simulink model "satellite_ADCS_pointing_simulation"  (R2022b)
settings: Solver=FixedStepAuto  StartTime=t0  StopTime=T_o  FixedStep=0.1  RelTol=1e-9  AbsTol=1e-9
values from neighbouring files (symbols this model uses):
  A0 = Af    [satellite_ADCS_LEOP_simulation.m]
  a0 = [adx0 ady0 adz0 ax0 ay0 az0]    [satellite_ADCS_LEOP_simulation.m]
  A_sb_1 = [999.999999992226e-003    3.46376307675883e-006   -1.88420189887425e-006 ... (first row only)    [satellite_ADCS_LEOP_simulation.m]
  A_sb_2 = [999.999999948501e-003   -10.1488410044293e-006   -22.0178875132149e-012 ... (first row only)    [satellite_ADCS_LEOP_simulation.m]
  A_sb_3 = [999.999999975613e-003   -46.6812699606578e-012    6.98384920637069e-006 ... (first row only)    [satellite_ADCS_LEOP_simulation.m]
  Ac = [0 (1-Ky)*n 0 -Ky*n^2 0 0 ... (first row only)    [satellite_ADCS_LEOP_simulation.m]
  alphaG_0 = pi/1.5    (= 2.09439510239)    [satellite_ADCS_LEOP_simulation.m]
  Bc = [J^-1; zeros(3,3)]    [satellite_ADCS_LEOP_simulation.m]
  Cc = [0 0 0 1 0 0 ... (first row only)    [satellite_ADCS_LEOP_simulation.m]
  Dc = zeros(3,3)    [satellite_ADCS_LEOP_simulation.m]
  E = 1    [satellite_ADCS_LEOP_simulation.m]
  F = 1e-3    (= 0.001)    [satellite_ADCS_LEOP_simulation.m]
  FOV = deg2rad(21.7)    [satellite_ADCS_LEOP_simulation.m]
  g_nm = S_matrix.*g_coefficients    [satellite_ADCS_LEOP_simulation.m]
  h_nm = S_matrix.*h_coefficients    [satellite_ADCS_LEOP_simulation.m]
  J = diag([Ix,Iy,Iz])    [satellite_ADCS_LEOP_simulation.m]
  J2 = 1.082e-3    (= 0.001082)    [satellite_ADCS_LEOP_simulation.m]
  K = lqry(SC,Qc,Rc)    [satellite_ADCS_LEOP_simulation.m]
  K_matrix = zeros(5,6)    [satellite_ADCS_LEOP_simulation.m]
  kep = [a e i OM om thf]    [satellite_ADCS_LEOP_simulation.m]
  L = Lt'    [satellite_ADCS_LEOP_simulation.m]
  LL = 1e-5    (= 1e-05)    [satellite_ADCS_LEOP_simulation.m]
  m = [0.37 0.32 0.28]    [satellite_ADCS_LEOP_simulation.m]
  mu = astroConstants(13)    [satellite_ADCS_LEOP_simulation.m]
  n_sun = 2*pi/T_y    (= 1.99238499086e-07)    [satellite_ADCS_LEOP_simulation.m]
  omega_e = 2*pi/T_e    (= 7.27220521664e-05)    [satellite_ADCS_LEOP_simulation.m]
  P00 = 1    [satellite_ADCS_LEOP_simulation.m]
  pR = pinv(R)    [satellite_ADCS_LEOP_simulation.m]
  R = [0 0 dz/2 0 0 -dz/2 ... (first row only)    [satellite_ADCS_LEOP_simulation.m]
  rt = astroConstants(23)    [satellite_ADCS_LEOP_simulation.m]
  S = S'    [satellite_ADCS_LEOP_simulation.m]
  sensor_noise = deg2rad(50/3600)    [satellite_ADCS_LEOP_simulation.m]
  sensor_sample_time = 1    [satellite_ADCS_LEOP_simulation.m]
  t0 = tf    (= 3200)    [satellite_ADCS_LEOP_simulation.m]
  T_o = 2*pi/n    [satellite_ADCS_LEOP_simulation.m]
  Te = 0.03    [satellite_ADCS_LEOP_simulation.m]
  Tp = [999.999926226686e-003    355.891478141766e-006   -144.526391847740e-006 ... (first row only)    [satellite_ADCS_LEOP_simulation.m]
  UL = 1e-4    (= 0.0001)    [satellite_ADCS_LEOP_simulation.m]
  w0 = wf    [satellite_ADCS_LEOP_simulation.m]
libraries: matrix_library x7, vrlib x3, sharedutil x2, aerolibutil x2
(part 2 of 3)

== system satellite_ADCS_pointing_simulation/SAD/Attitude Determination ==
  note: matrix of star catalogue in inertial frame
  note: Star Sampling & Attitude Determination
  note: s/c attitude
  S_n : Inport
  w : Inport  Port=2
  A_b/n : Inport  Port=3
  Algebraic Attitude Determination : Subsystem  Commented=on
      settings: PortSchema="{\"entries\":[{\"content\":{\"sides\":[{\"content\":{\"connectorIds\":[\"In1\",\"In2\"]},\"type\":\"ConnectorPlacement.EquallySpacedRectSide\",\"uuid\":\"6504138f-2a85-4d38-9815-f5cddec5de59\"},{\"content\":{\"connectorIds\":[\"Out1\"],\"side\":\"RIGHT\"},\"type\":\"ConnectorPlacement.EquallySpacedRectSide\",\"uuid\":\"322c0af4-c8eb-4770-b746-148ad674ab50\"},{\"content\":{\"connectorIds\":[\"In3\"],\"side\":\"TOP\"},\"type\":\"ConnectorPlacement.EquallySpacedRectSide\",\"uuid\":\"b986788c-e235-4c96-906b-8e6936550346\"}]},\"type\":\"ConnectorPlacement.EquallySpacedConnector\",\"uuid\":\"9dab80e4-0566-4f6e-b7d4-73f1fb3580cf\"}],\"packageUris\":[\"http://schema.mathworks.com/mf0/Connector/R2020b\"],\"version\":\"1.0\"}"
  Constant3 : Constant  Value=S
  Demux : Demux  Outputs=3
  Scope : Scope
  Sensor1 xpos : Subsystem
  Sensor2 ypos : Subsystem
  Sensor3 zpos : Subsystem
  Sun Sensors : Subsystem
  Vector Concatenate2 : Concatenate  Commented=on  NumInputs=3  Mode=Multidimensional array  ConcatenateDimension=2
  Vector Concatenate3 : Concatenate  Commented=on  NumInputs=3  Mode=Multidimensional array  ConcatenateDimension=2
  Wabha Attitude Determination : Subsystem
      settings: PortSchema="{\"entries\":[{\"content\":{\"sides\":[{\"content\":{\"connectorIds\":[\"In1\",\"In2\",\"In3\",\"In4\",\"In5\",\"In6\"]},\"type\":\"ConnectorPlacement.EquallySpacedRectSide\",\"uuid\":\"d5b8c53a-8fd4-43f2-87af-7adc7e94ab2c\"},{\"content\":{\"connectorIds\":[\"Out1\"],\"side\":\"RIGHT\"},\"type\":\"ConnectorPlacement.EquallySpacedRectSide\",\"uuid\":\"9cba7d00-4c67-4fcd-90db-1f4702b8291d\"},{\"content\":{\"connectorIds\":[\"In7\"],\"side\":\"TOP\"},\"type\":\"ConnectorPlacement.EquallySpacedRectSide\",\"uuid\":\"005be892-b0ea-47ef-a10a-03c751d6d0c9\"}]},\"type\":\"ConnectorPlacement.EquallySpacedConnector\",\"uuid\":\"48132ded-170f-499d-b299-faa3505412b0\"}],\"packageUris\":[\"http://schema.mathworks.com/mf0/Connector/R2020b\"],\"version\":\"1.0\"}"
  Zero-Order Hold : ZeroOrderHold  SampleTime=sensor_sample_time
  Zero-Order Hold1 : ZeroOrderHold  SampleTime=sensor_sample_time
  A*_b/n : Outport
  wires:
  Wabha Attitude Determination/1(A*_b/n) -> Scope/1, A*_b/n/1
  Sensor3 zpos/2(v3) -> Wabha Attitude Determination/6(v3)
  Sensor3 zpos/1(s3) -> Wabha Attitude Determination/5(s3)
  Sensor2 ypos/2(v2) -> Wabha Attitude Determination/4(v2)
  Sensor2 ypos/1(s2) -> Wabha Attitude Determination/3(s2)
  Sensor1 xpos/2(v1) -> Wabha Attitude Determination/2(v1)
  Sensor1 xpos/1(s1) -> Wabha Attitude Determination/1(s1)
  Zero-Order Hold1/1 -> Sun Sensors/1(S_n)
  Sun Sensors/1(Sun Obstruction) -> Demux/1, Wabha Attitude Determination/7(E)  "E"
  S_n/1 -> Zero-Order Hold1/1
  Demux/1 -> Sensor1 xpos/Enable
  Demux/2 -> Sensor2 ypos/Enable
  Demux/3 -> Sensor3 zpos/Enable
  Vector Concatenate2/1 -> Algebraic Attitude Determination/2(V)  "V"
  Vector Concatenate3/1 -> Algebraic Attitude Determination/1(S)  "S"
  Constant3/1 -> Sensor1 xpos/3(S), Sensor2 ypos/3(S), Sensor3 zpos/3(S)
  A_b/n/1 -> Zero-Order Hold/1
  Zero-Order Hold/1 -> Sun Sensors/2(A_b/n), Sensor1 xpos/2(A_b/n), Sensor2 ypos/2(A_b/n), Sensor3 zpos/2(A_b/n)
  w/1 -> Sensor2 ypos/1(w), Sensor1 xpos/1(w), Sensor3 zpos/1(w)

== system satellite_ADCS_pointing_simulation/SAD/Control Parameters ==
  A_l/n : Inport
  A*_b/n : Inport  Port=2
  . : Product  Multiplication=Matrix(*)
  Display : Display
  Gain : Gain  Gain=1/2
  Gain1 : Gain  Gain=1/2
  Gain2 : Gain  Gain=1/2
  Gain3 : Gain  Gain=180/pi
  Gain4 : Gain  Gain=180/pi
  Gain5 : Gain  Gain=180/pi
  Mux : Mux  Inputs=3
  Mux1 : Mux  Inputs=3
  Scope : Scope  NumInputPorts=3
  Selector : Selector  NumberOfDimensions=2  InputPortWidth=3  IndexOptions=Index vector (dialog),Index vector (dialog)  Indices=1,3  OutputSizes=1,1
  Selector1 : Selector  NumberOfDimensions=2  InputPortWidth=3  IndexOptions=Index vector (dialog),Index vector (dialog)  Indices=1,2  OutputSizes=1,1
  Selector2 : Selector  NumberOfDimensions=2  InputPortWidth=3  IndexOptions=Index vector (dialog),Index vector (dialog)  Indices=2,1  OutputSizes=1,1
  Selector3 : Selector  NumberOfDimensions=2  InputPortWidth=3  IndexOptions=Index vector (dialog),Index vector (dialog)  Indices=3,2  OutputSizes=1,1
  Selector4 : Selector  NumberOfDimensions=2  InputPortWidth=3  IndexOptions=Index vector (dialog),Index vector (dialog)  Indices=2,3  OutputSizes=1,1
  Selector5 : Selector  NumberOfDimensions=2  InputPortWidth=3  IndexOptions=Index vector (dialog),Index vector (dialog)  Indices=3,1  OutputSizes=1,1
  Subtract1 : Sum  Inputs=+-
  Subtract2 : Sum  Inputs=+-
  Subtract3 : Sum  Inputs=+-
  To Workspace : ToWorkspace  VariableName=alphas  SampleTime=0.1
  Transpose : Math  Operator=transpose
  Zero-Order Hold : ZeroOrderHold  SampleTime=sensor_sample_time
  y^ : Outport
  wires:
  A_l/n/1 -> Zero-Order Hold/1
  Zero-Order Hold/1 -> Transpose/1
  Transpose/1 -> ./2  "A_n/l"
  A*_b/n/1 -> ./1
  ./1 -> Selector2/1, Selector1/1, Selector/1, Selector4/1, Display/1, Selector3/1, Selector5/1  "Ae"
  Selector5/1 -> Subtract1/1  "a31"
  Selector/1 -> Subtract1/2  "a13"
  Selector1/1 -> Subtract2/1  "a12"
  Selector2/1 -> Subtract2/2  "a21"
  Subtract1/1 -> Gain/1
  Subtract2/1 -> Gain1/1
  Mux/1 -> y^/1
  Subtract3/1 -> Gain2/1
  Selector3/1 -> Subtract3/2  "a32"
  Selector4/1 -> Subtract3/1  "a23"
  Gain3/1 -> Scope/1
  Gain4/1 -> Scope/2
  Gain5/1 -> Scope/3
  Gain/1 -> Mux1/2, Gain4/1, Mux/2  "ay"
  Gain2/1 -> Mux1/1, Mux/1, Gain3/1  "ax"
  Gain1/1 -> Mux1/3, Gain5/1, Mux/3  "az"
  Mux1/1 -> To Workspace/1

== system satellite_ADCS_pointing_simulation/Actuators/Logic Switch F1/Enabled Subsystem ==
  In1 : Inport
  Enable : EnablePort
  Constant1 : Constant
  GreaterThan : RelationalOperator  OutDataTypeStr=boolean  RndMeth=Simplest  InputSameDT=off
  LL : Constant  Value=LL
  e : Outport
  y : Outport  Port=2
  wires:
  In1/1 -> GreaterThan/1
  GreaterThan/1 -> e/1
  LL/1 -> GreaterThan/2
  Constant1/1 -> y/1

== system satellite_ADCS_pointing_simulation/Actuators/Logic Switch F1/Enabled Subsystem1 ==
  In1 : Inport
  Enable : EnablePort
  Constant1 : Constant  Value=0
  GreaterThan : RelationalOperator  OutDataTypeStr=boolean  RndMeth=Simplest  InputSameDT=off
  UL : Constant  Value=UL
  e : Outport
  y : Outport  Port=2
  wires:
  UL/1 -> GreaterThan/2
  In1/1 -> GreaterThan/1
  GreaterThan/1 -> e/1
  Constant1/1 -> y/1

== system satellite_ADCS_pointing_simulation/Actuators/Logic Switch F2/Enabled Subsystem ==
  In1 : Inport
  Enable : EnablePort
  Constant1 : Constant
  GreaterThan : RelationalOperator  OutDataTypeStr=boolean  RndMeth=Simplest  InputSameDT=off
  LL : Constant  Value=LL
  e : Outport
  y : Outport  Port=2
  wires:
  Constant1/1 -> y/1
  LL/1 -> GreaterThan/2
  GreaterThan/1 -> e/1
  In1/1 -> GreaterThan/1

== system satellite_ADCS_pointing_simulation/Actuators/Logic Switch F2/Enabled Subsystem1 ==
  In1 : Inport
  Enable : EnablePort
  Constant1 : Constant  Value=0
  GreaterThan : RelationalOperator  OutDataTypeStr=boolean  RndMeth=Simplest  InputSameDT=off
  UL : Constant  Value=UL
  e : Outport
  y : Outport  Port=2
  wires:
  Constant1/1 -> y/1
  GreaterThan/1 -> e/1
  In1/1 -> GreaterThan/1
  UL/1 -> GreaterThan/2

== system satellite_ADCS_pointing_simulation/Actuators/Logic Switch F3/Enabled Subsystem ==
  In1 : Inport
  Enable : EnablePort
  Constant1 : Constant
  GreaterThan : RelationalOperator  OutDataTypeStr=boolean  RndMeth=Simplest  InputSameDT=off
  LL : Constant  Value=LL
  e : Outport
  y : Outport  Port=2
  wires:
  In1/1 -> GreaterThan/1
  GreaterThan/1 -> e/1
  LL/1 -> GreaterThan/2
  Constant1/1 -> y/1

== system satellite_ADCS_pointing_simulation/Actuators/Logic Switch F3/Enabled Subsystem1 ==
  In1 : Inport
  Enable : EnablePort
  Constant1 : Constant  Value=0
  GreaterThan : RelationalOperator  OutDataTypeStr=boolean  RndMeth=Simplest  InputSameDT=off
  UL : Constant  Value=UL
  e : Outport
  y : Outport  Port=2
  wires:
  UL/1 -> GreaterThan/2
  In1/1 -> GreaterThan/1
  GreaterThan/1 -> e/1
  Constant1/1 -> y/1

== system satellite_ADCS_pointing_simulation/Actuators/Logic Switch F4/Enabled Subsystem ==
  In1 : Inport
  Enable : EnablePort
  Constant1 : Constant
  GreaterThan : RelationalOperator  OutDataTypeStr=boolean  RndMeth=Simplest  InputSameDT=off
  LL : Constant  Value=LL
  e : Outport
  y : Outport  Port=2
  wires:
  Constant1/1 -> y/1
  LL/1 -> GreaterThan/2
  GreaterThan/1 -> e/1
  In1/1 -> GreaterThan/1

== system satellite_ADCS_pointing_simulation/Actuators/Logic Switch F4/Enabled Subsystem1 ==
  In1 : Inport
  Enable : EnablePort
  Constant1 : Constant  Value=0
  GreaterThan : RelationalOperator  OutDataTypeStr=boolean  RndMeth=Simplest  InputSameDT=off
  UL : Constant  Value=UL
  e : Outport
  y : Outport  Port=2
  wires:
  Constant1/1 -> y/1
  GreaterThan/1 -> e/1
  In1/1 -> GreaterThan/1
  UL/1 -> GreaterThan/2

== system satellite_ADCS_pointing_simulation/Actuators/Logic Switch F5/Enabled Subsystem ==
  In1 : Inport
  Enable : EnablePort
  Constant1 : Constant
  GreaterThan : RelationalOperator  OutDataTypeStr=boolean  RndMeth=Simplest  InputSameDT=off
  LL : Constant  Value=LL
  e : Outport
  y : Outport  Port=2
  wires:
  In1/1 -> GreaterThan/1
  GreaterThan/1 -> e/1
  LL/1 -> GreaterThan/2
  Constant1/1 -> y/1

== system satellite_ADCS_pointing_simulation/Actuators/Logic Switch F5/Enabled Subsystem1 ==
  In1 : Inport
  Enable : EnablePort
  Constant1 : Constant  Value=0
  GreaterThan : RelationalOperator  OutDataTypeStr=boolean  RndMeth=Simplest  InputSameDT=off
  UL : Constant  Value=UL
  e : Outport
  y : Outport  Port=2
  wires:
  UL/1 -> GreaterThan/2
  In1/1 -> GreaterThan/1
  GreaterThan/1 -> e/1
  Constant1/1 -> y/1

== system satellite_ADCS_pointing_simulation/Actuators/Logic Switch F6/Enabled Subsystem ==
  In1 : Inport
  Enable : EnablePort
  Constant1 : Constant
  GreaterThan : RelationalOperator  OutDataTypeStr=boolean  RndMeth=Simplest  InputSameDT=off
  LL : Constant  Value=LL
  e : Outport
  y : Outport  Port=2
  wires:
  Constant1/1 -> y/1
  LL/1 -> GreaterThan/2
  GreaterThan/1 -> e/1
  In1/1 -> GreaterThan/1

== system satellite_ADCS_pointing_simulation/Actuators/Logic Switch F6/Enabled Subsystem1 ==
  In1 : Inport
  Enable : EnablePort
  Constant1 : Constant  Value=0
  GreaterThan : RelationalOperator  OutDataTypeStr=boolean  RndMeth=Simplest  InputSameDT=off
  UL : Constant  Value=UL
  e : Outport
  y : Outport  Port=2
  wires:
  Constant1/1 -> y/1
  GreaterThan/1 -> e/1
  In1/1 -> GreaterThan/1
  UL/1 -> GreaterThan/2

== system satellite_ADCS_pointing_simulation/Disturbance Torques/Local S//C Frame/R1(i) ==
  a : Inport
  Add : Sum  Inputs=+++
  Constant : Constant  Value=[0 0 0; 0 1 0; 0 0 1]
  Constant1 : Constant  Value=[0 0 0; 0 0 1; 0 -1 0]
  Constant2 : Constant  Value=[1 0 0; 0 0 0; 0 0 0]
  Cos : Trigonometry  Operator=cos
  Product : Product
  Product1 : Product
  Sin : Trigonometry
  R1 : Outport
  wires:
  a/1 -> Cos/1, Sin/1
  Cos/1 -> Product/2
  Constant/1 -> Product/1
  Constant1/1 -> Product1/1
  Sin/1 -> Product1/2
  Product/1 -> Add/1
  Constant2/1 -> Add/3
  Product1/1 -> Add/2
  Add/1 -> R1/1

== system satellite_ADCS_pointing_simulation/Disturbance Torques/Local S//C Frame/R3(OM) ==
  a : Inport
  Add : Sum  Inputs=+++
  Constant : Constant  Value=[1 0 0; 0 1 0; 0 0 0]
  Constant1 : Constant  Value=[0 1 0; -1 0 0; 0 0 0]
  Constant2 : Constant  Value=[0 0 0; 0 0 0; 0 0 1]
  Cos : Trigonometry  Operator=cos
  Product : Product
  Product1 : Product
  Sin : Trigonometry
  R3 : Outport
  wires:
  a/1 -> Cos/1, Sin/1
  Cos/1 -> Product/2
  Constant/1 -> Product/1
  Constant1/1 -> Product1/1
  Sin/1 -> Product1/2
  Product/1 -> Add/1
  Constant2/1 -> Add/3
  Product1/1 -> Add/2
  Add/1 -> R3/1

== system satellite_ADCS_pointing_simulation/Disturbance Torques/Local S//C Frame/R3(om+th) ==
  a : Inport
  Add : Sum  Inputs=+++
  Constant : Constant  Value=[1 0 0; 0 1 0; 0 0 0]
  Constant1 : Constant  Value=[0 1 0; -1 0 0; 0 0 0]
  Constant2 : Constant  Value=[0 0 0; 0 0 0; 0 0 1]
  Cos : Trigonometry  Operator=cos
  Product : Product
  Product1 : Product
  Sin : Trigonometry
  R3 : Outport
  wires:
  a/1 -> Cos/1, Sin/1
  Cos/1 -> Product/2
  Constant/1 -> Product/1
  Constant1/1 -> Product1/1
  Sin/1 -> Product1/2
  Product/1 -> Add/1
  Constant2/1 -> Add/3
  Product1/1 -> Add/2
  Add/1 -> R3/1

== system satellite_ADCS_pointing_simulation/Disturbance Torques/Local S//C Frame/RAAN Precession ==
  p : Inport
  i : Inport  Port=2
  Enable : EnablePort
  Clock1 : Clock
  Constant8 : Constant  Value=rt
  Constant9 : Constant  Value=J2
  Cos : Trigonometry  Operator=cos
  Divide3 : Product  Inputs=*/
  Gain : Gain  Gain=-3*pi
  Gain1 : Gain  Gain=T_o
  Product1 : Product  Inputs=3
  Product6 : Product
  Square1 : Math  Operator=square
  Square2 : Math  Operator=square
  D_OM : Outport
  wires:
  Cos/1 -> Product1/3
  Square1/1 -> Gain1/1  "p^2"
  Gain/1 -> Divide3/1
  Constant9/1 -> Product1/1
  Clock1/1 -> Product6/2
  Product1/1 -> Gain/1
  p/1 -> Square1/1
  Gain1/1 -> Divide3/2
  Divide3/1 -> Product6/1
  Square2/1 -> Product1/2
  Constant8/1 -> Square2/1
  i/1 -> Cos/1
  Product6/1 -> D_OM/1

== system satellite_ADCS_pointing_simulation/Disturbance Torques/Local S//C Frame/RAAN Precession Switch ==
  Constant : Constant
  Constant1 : Constant  Value=0
  Off : Outport
  On : Outport  Port=2
  wires:
  Constant/1 -> On/1
  Constant1/1 -> Off/1

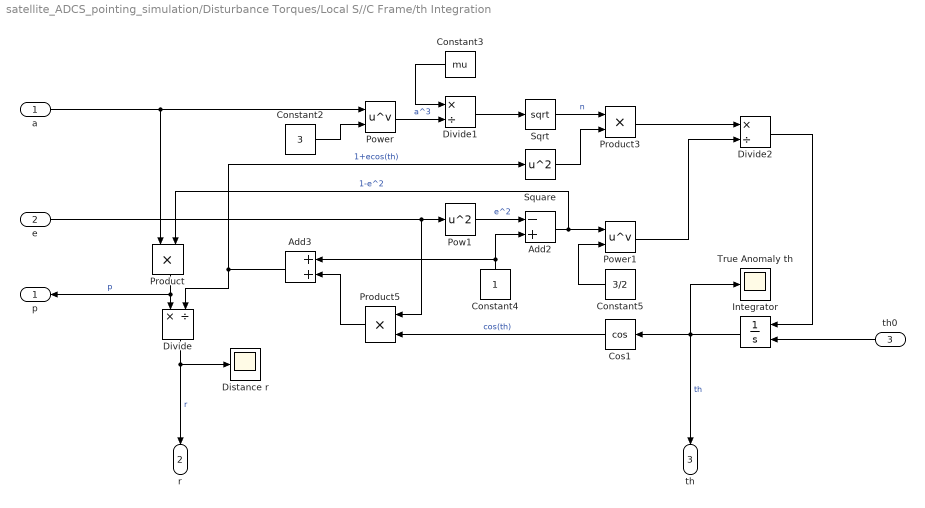
== system satellite_ADCS_pointing_simulation/Disturbance Torques/Local S//C Frame/th Integration ==
  a : Inport
  e : Inport  Port=2
  th0 : Inport  Port=3
  Add2 : Sum  Inputs=-+
  Add3 : Sum
  Constant2 : Constant  Value=3
  Constant3 : Constant  Value=mu
  Constant4 : Constant
  Constant5 : Constant  Value=3/2
  Cos1 : Trigonometry  Operator=cos
  Distance r : Scope
  Divide : Product  Inputs=*/
  Divide1 : Product  Inputs=*/
  Divide2 : Product  Inputs=*/
  Integrator : Integrator  InitialConditionSource=external  WrapState=on  WrappedStateUpperValue=2*pi  WrappedStateLowerValue=0
  Pow1 : Math  Operator=square  SignedPower=on  RndMeth=Zero
  Power : Math  Operator=pow
  Power1 : Math  Operator=pow
  Product : Product
  Product3 : Product
  Product5 : Product
  Sqrt : Sqrt
  Square : Math  Operator=square
  True Anomaly th : Scope
  p : Outport
  r : Outport  Port=2
  th : Outport  Port=3
  wires:
  Constant5/1 -> Power1/2
  Cos1/1 -> Product5/2  "cos(th)"
  Divide/1 -> Distance r/1, r/1  "r"
  Power/1 -> Divide1/2  "a^3"
  Constant4/1 -> Add2/2, Add3/1
  a/1 -> Product/1, Power/1
  e/1 -> Product5/1, Pow1/1
  Square/1 -> Product3/2
  Sqrt/1 -> Product3/1  "n"
  Add2/1 -> Power1/1, Product/2  "1-e^2"
  Divide1/1 -> Sqrt/1
  Product3/1 -> Divide2/1
  Pow1/1 -> Add2/1  "e^2"
  Add3/1 -> Divide/2, Square/1  "1+ecos(th)"
  Constant2/1 -> Power/2
  Constant3/1 -> Divide1/1
  Integrator/1 -> Cos1/1, True Anomaly th/1, th/1  "th"
  Product/1 -> p/1, Divide/1  "p"
  Divide2/1 -> Integrator/1
  Product5/1 -> Add3/2
  Power1/1 -> Divide2/2
  th0/1 -> Integrator/2

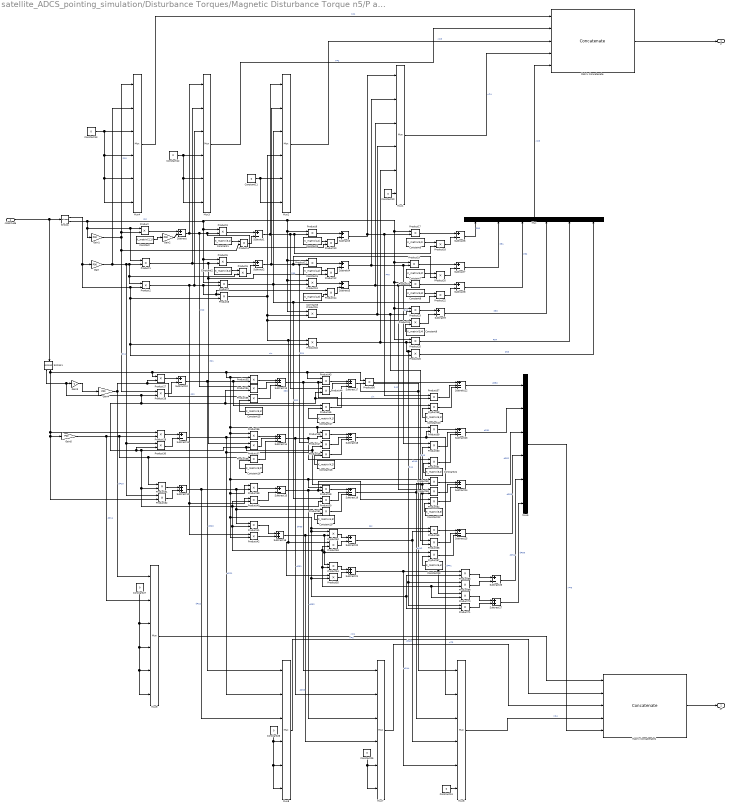
== system satellite_ADCS_pointing_simulation/Disturbance Torques/Magnetic Disturbance Torque n5/P and dP matrices ==
  colatitude : Inport
  Constant : Constant  Value=K_matrix(2,1)
  Constant1 : Constant  Value=K_matrix(3,1)
  Constant{10..13,24..27} (8 alike) : Constant  Value=0
  Constant15 : Constant  Value=K_matrix(3,1)
  Constant16 : Constant  Value=K_matrix(3,2)
  Constant17 : Constant  Value=K_matrix(4,1)
  Constant18 : Constant  Value=K_matrix(4,2)
  Constant19 : Constant  Value=K_matrix(4,3)
  Constant2 : Constant  Value=K_matrix(3,2)
  Constant20 : Constant  Value=K_matrix(5,1)
  Constant21 : Constant  Value=K_matrix(5,2)
  Constant22 : Constant  Value=K_matrix(5,3)
  Constant23 : Constant  Value=K_matrix(5,4)
  Constant3 : Constant  Value=K_matrix(4,1)
  Constant4 : Constant  Value=K_matrix(4,2)
  Constant5 : Constant  Value=K_matrix(4,3)
  Constant6 : Constant  Value=K_matrix(5,1)
  Constant7 : Constant  Value=K_matrix(5,2)
  Constant8 : Constant  Value=K_matrix(5,3)
  Constant9 : Constant  Value=K_matrix(5,4)
  Gain{,1..2,4..5} (5 alike) : Gain  Gain=P00
  Gain3 : Gain  Gain=-1
  Matrix Concatenate : Concatenate  NumInputs=5  Mode=Multidimensional array  ConcatenateDimension=2
  Matrix Concatenate1 : Concatenate  NumInputs=5  Mode=Multidimensional array  ConcatenateDimension=2
  Mux{,1..9} (10 alike) : Mux  Inputs=6
  Product{,1..71} (72 alike) : Product
  SinCos : Trigonometry  Operator=sincos
  SinCos1 : Trigonometry  Operator=sincos
  Subtract{,1..11,15,20,26} (15 alike) : Sum  Inputs=+-
  Subtract{12,16,21,27} (4 alike) : Sum
  Subtract{13..14,17..19,22..25} (9 alike) : Sum  Inputs=+--
  P : Outport
  dP : Outport  Port=2
  wires:
  SinCos1/2 -> Product39/1, Product65/1, Product52/1, Product55/2, Product68/2, Product71/2, Product42/2, Product62/1, Product49/1, Product36/1, Product59/1, Product46/1, Product33/1, Product56/1, Product43/1, Product27/1, Product32/2, Gain5/1, Product29/1  "cos"
  Subtract19/1 -> Mux6/3, Product62/2  "dP42"
  Product2/1 -> Product40/1, Product42/1, Mux3/3, Product14/1, Product8/1, Product7/2  "P22"
  Constant27/1 -> Mux9/4, Mux9/5, Mux9/6, Mux9/3
  Subtract24/1 -> Mux5/3  "dP52"
  Product28/1 -> Subtract10/2
  Constant13/1 -> Mux4/6, Mux4/5, Mux4/4, Mux4/3
  Product58/1 -> Subtract22/3
  Product45/1 -> Subtract17/3
  Product49/1 -> Subtract19/1
  Constant8/1 -> Product22/1
  SinCos/2 -> Product25/1, Product23/1, Product21/1, Product19/1, Product17/1, Product15/1, Product13/1, Product11/1, Product9/1, Product7/1, Product5/1, Product3/1, Gain1/1, Product1/1, Product/1  "cos"
  Subtract18/1 -> Mux6/2, Product59/2  "dP41"
  Product62/1 -> Subtract24/1
  Product66/1 -> Subtract25/2
  Subtract21/1 -> Mux6/5, Product70/1, Product68/1  "dP44"
  SinCos1/1 -> Product44/2, Product57/2, Product34/2, Product54/2, Product70/2, Product69/2, Product53/2, Product41/2, Product50/2, Product40/2, Product31/2, Product47/2, Product66/2, Product63/2, Product60/2, Product37/2, Product30/2, Product28/2, Gain3/1  "sin"
  Product46/1 -> Subtract18/1
  Subtract7/1 -> Mux/2  "P51"
  Product1/1 -> Mux3/2, Product37/1, Product12/2, Product5/2  "P21"
  Constant20/1 -> Product58/2
  Mux4/1 -> Matrix Concatenate/1  "n=1"
  Gain5/1 -> Mux9/2, Product31/1, Product38/1, Product29/2  "dP11"
  Product8/1 -> Mux2/4, Product55/1, Product53/1, Product16/1, Product24/1, Product15/2  "P33"
  Product60/1 -> Subtract23/2
  Product15/1 -> Product66/1, Product23/2, Mux1/4  "P43"
  Product7/1 -> Mux2/3, Product13/2, Product50/1, Product22/2  "P32"
  SinCos/1 -> Product8/2, Product26/2, Product16/2, Product2/2, Gain/1  "sin"
  Mux5/1 -> Matrix Concatenate1/5  "n=5"
  colatitude/1 -> SinCos1/1, SinCos/1
  Constant12/1 -> Mux3/5, Mux3/6, Mux3/4
  Product10/1 -> Subtract3/2
  Constant4/1 -> Product12/1
  Gain1/1 -> Product28/1, Product4/2, Mux4/1, Product/2  "P10"
  Product50/1 -> Subtract19/2
  Constant19/1 -> Product51/2
  Subtract12/1 -> Mux8/3, Product41/1, Product51/1, Product39/2  "dP22"
  Mux2/1 -> Matrix Concatenate/3  "n=3"
  Gain/1 -> Product32/1, Product30/1, Product2/1, Product6/2, Product1/2, Mux4/2  "P11"
  Constant5/1 -> Product14/2
  Constant6/1 -> Product18/1
  Constant2/1 -> Product6/1
  Gain2/1 -> Subtract/2
  Constant/1 -> Gain2/1
  Gain3/1 -> Gain4/1
  Constant22/1 -> Product64/2
  Product40/1 -> Subtract15/2
  Product4/1 -> Subtract1/2
  Mux3/1 -> Matrix Concatenate/2  "n=2"
  Subtract17/1 -> Mux6/1, Product56/2  "dP40"
  Mux7/1 -> Matrix Concatenate1/3  "n=3"
  Product68/1 -> Subtract26/1
  Product29/1 -> Subtract11/1
  Product16/1 -> Mux1/5, Product25/2, Product26/1, Product71/1, Product69/1  "P44"
  Subtract5/1 -> Mux1/3, Product63/1, Product21/2  "P42"
  Product/1 -> Subtract/1
  Matrix Concatenate1/1 -> dP/1
  Product41/1 -> Subtract16/1
  Subtract4/1 -> Product19/2, Product60/1, Mux1/2  "P41"
  Product5/1 -> Subtract2/1
  Product20/1 -> Subtract7/2
  Product6/1 -> Subtract2/2
  Constant3/1 -> Product10/1
  Subtract25/1 -> Mux5/4  "dP53"
  Constant16/1 -> Product38/2
  Subtract15/1 -> Mux7/3, Product64/1, Product49/2  "dP32"
  Gain4/1 -> Product35/1, Product27/2, Mux9/1  "dP10"
  Product65/1 -> Subtract25/1
  Subtract16/1 -> Product54/1, Product67/1, Product52/2, Mux7/4  "dP33"
  Product30/1 -> Subtract11/2
  Subtract13/1 -> Mux7/1, Product43/2, Product58/1  "dP30"
  Subtract1/1 -> Mux2/1, Product44/1, Product18/2, Product9/2  "P30"
  Subtract20/1 -> Mux6/4, Product65/2  "dP43"
  Product63/1 -> Subtract24/2
  Product53/1 -> Subtract20/2
  Product13/1 -> Subtract5/1
  Subtract27/1 -> Mux5/6  "dP55"
  Constant26/1 -> Mux8/6, Mux8/5, Mux8/4
  Constant24/1 -> Mux6/6
  Subtract14/1 -> Product46/2, Product61/1, Mux7/2  "dP31"
  Product22/1 -> Subtract8/2
  Subtract23/1 -> Mux5/2  "dP51"
  Subtract26/1 -> Mux5/5  "dP54"
  Constant18/1 -> Product48/2
  Mux8/1 -> Matrix Concatenate1/2  "n=2"
  Subtract/1 -> Mux3/1, Product34/1, Product10/2, Product3/2  "P20"
  Subtract3/1 -> Mux1/1, Product57/1, Product17/2  "P40"
  Product55/1 -> Subtract21/2
  Constant21/1 -> Product61/2
  Product18/1 -> Subtract6/2
  Constant11/1 -> Mux2/6, Mux2/5
  Product12/1 -> Subtract4/2
  Subtract2/1 -> Mux2/2, Product11/2, Product47/1, Product20/2  "P31"
  Product42/1 -> Subtract16/2
  Subtract9/1 -> Mux/4  "P53"
  Product19/1 -> Subtract7/1
  Subtract8/1 -> Mux/3  "P52"
  Constant10/1 -> Mux1/6
  Product11/1 -> Subtract4/1
  Product48/1 -> Subtract18/3
  Subtract10/1 -> Mux8/1, Product45/1, Product33/2  "dP20"
  Matrix Concatenate/1 -> P/1
  Constant17/1 -> Product45/2
  Constant15/1 -> Product35/2
  Product17/1 -> Subtract6/1
  Product3/1 -> Subtract1/1
  Product34/1 -> Subtract13/2
  Product25/1 -> Mux/5  "P54"
  Product14/1 -> Subtract5/2
  Constant23/1 -> Product67/2
  Product44/1 -> Subtract17/2
  Product57/1 -> Subtract22/2
  Product36/1 -> Subtract14/1
  Constant7/1 -> Product20/1
  Constant1/1 -> Product4/1
  Product24/1 -> Subtract9/2
  Product9/1 -> Subtract3/1
  Mux1/1 -> Matrix Concatenate/4  "n=4"
  Subtract6/1 -> Mux/1  "P50"
  Product27/1 -> Subtract10/1
  Product23/1 -> Subtract9/1
  Constant9/1 -> Product24/2
  Product21/1 -> Subtract8/1
  Product56/1 -> Subtract22/1
  Product47/1 -> Subtract18/2
  Product26/1 -> Mux/6  "P55"
  Product51/1 -> Subtract19/3
  Product43/1 -> Subtract17/1
  Product35/1 -> Subtract13/3
  Product31/1 -> Subtract12/1
  Mux/1 -> Matrix Concatenate/5  "n=5"
  Subtract22/1 -> Mux5/1  "dP50"
  Product59/1 -> Subtract23/1
  Product33/1 -> Subtract13/1
  Product38/1 -> Subtract14/3
  Product37/1 -> Subtract14/2
  Product32/1 -> Subtract12/2
  Subtract11/1 -> Product48/1, Mux8/2, Product36/2  "dP21"
  Product54/1 -> Subtract21/1
  Constant25/1 -> Mux7/6, Mux7/5
  Product39/1 -> Subtract15/1
  Product61/1 -> Subtract23/3
  Product52/1 -> Subtract20/1
  Product64/1 -> Subtract24/3
  Product71/1 -> Subtract27/2
  Product69/1 -> Subtract26/2
  Mux6/1 -> Matrix Concatenate1/4  "n=4"
  Product67/1 -> Subtract25/3
  Product70/1 -> Subtract27/1
  Mux9/1 -> Matrix Concatenate1/1  "n=1"

== system satellite_ADCS_pointing_simulation/Disturbance Torques/Magnetic Disturbance Torque n5/Subsystem ==
  note: right ascension
  note: declination
  r_n : Inport
  Asin : Trigonometry  Operator=asin
  Atan2 : Trigonometry  Operator=atan2
  Clock1 : Clock
  Constant1 : Constant  Value=alphaG_0
  Constant2 : Constant  Value=pi/2
  Demux : Demux  Outputs=3
  Divide1 : Product  Inputs=*/
  Dot Product1 : DotProduct  OutDataTypeStr=Inherit: Inherit via internal rule
  Gain : Gain  Gain=omega_e
  Sqrt : Sqrt
  Subtract : Sum  Inputs=|++
  Subtract1 : Sum  Inputs=+-
  Subtract2 : Sum  Inputs=-+
  r : Outport
  Longitude : Outport  Port=2
  RA : Outport  Port=3
  DELTA : Outport  Port=4
  Colatitude : Outport  Port=5
  wires:
  Atan2/1 -> Subtract1/1, RA/1  "alpha RA"
  Divide1/1 -> Asin/1
  Clock1/1 -> Gain/1
  Sqrt/1 -> r/1, Divide1/2  "Distance From Earth"
  Asin/1 -> Subtract2/1, DELTA/1
  Demux/2 -> Atan2/1  "y"
  Gain/1 -> Subtract/1
  Dot Product1/1 -> Sqrt/1
  Demux/1 -> Atan2/2  "x"
  r_n/1 -> Dot Product1/1, Dot Product1/2, Demux/1
  Constant1/1 -> Subtract/2
  Demux/3 -> Divide1/1  "z"
  Subtract2/1 -> Colatitude/1  "Colatitude THETA"
  Subtract/1 -> Subtract1/2  "th_Greenwich"
  Subtract1/1 -> Longitude/1
  Constant2/1 -> Subtract2/2

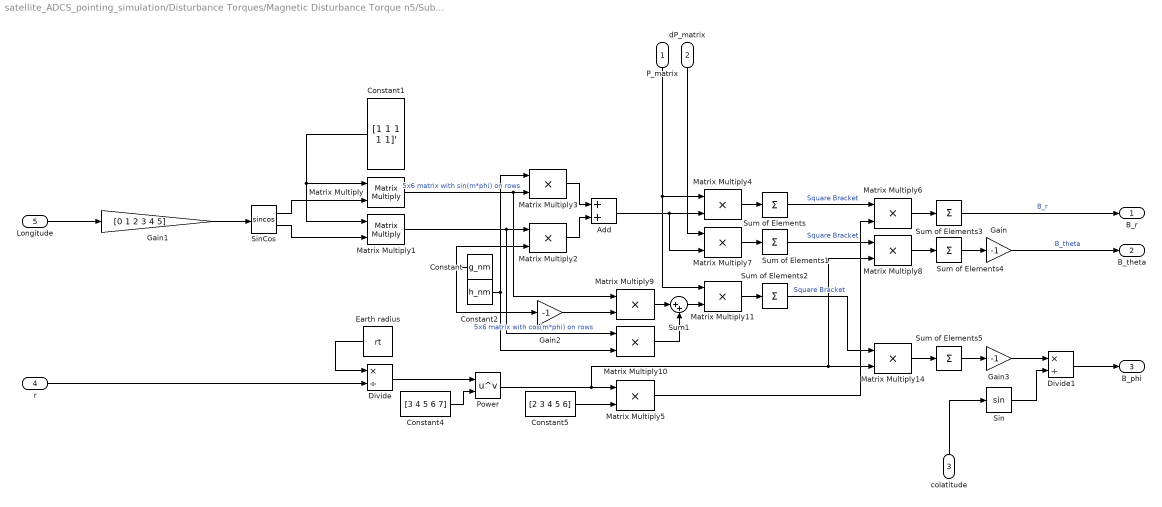
== system satellite_ADCS_pointing_simulation/Disturbance Torques/Magnetic Disturbance Torque n5/Subsystem1 ==
  P_matrix : Inport
  dP_matrix : Inport  Port=2
  colatitude : Inport  Port=3
  r : Inport  Port=4
  Longitude : Inport  Port=5
  Add : Sum
  Constant : Constant  Value=g_nm
  Constant1 : Constant  Value=[1 1 1 1 1]'  VectorParams1D=off
  Constant2 : Constant  Value=h_nm
  Constant4 : Constant  Value=[3 4 5 6 7]
  Constant5 : Constant  Value=[2 3 4 5 6]
  Divide : Product  Inputs=*/
  Divide1 : Product  Inputs=*/
  Earth radius : Constant  Value=rt
  Gain : Gain  Gain=-1
  Gain1 : Gain  Gain=[0 1 2 3 4 5]
  Gain2 : Gain  Gain=-1
  Gain3 : Gain  Gain=-1
  Matrix Multiply : Product  Multiplication=Matrix(*)
  Matrix Multiply1 : Product  Multiplication=Matrix(*)
  Matrix Multiply{2..11,14} (11 alike) : Product
  Power : Math  Operator=pow
  Sin : Trigonometry
  SinCos : Trigonometry  Operator=sincos
  Sum of Elements : Sum  Inputs=+  CollapseMode=Specified dimension  CollapseDim=2
  Sum of Elements1 : Sum  Inputs=+  CollapseMode=Specified dimension  CollapseDim=2
  Sum of Elements2 : Sum  Inputs=+  CollapseMode=Specified dimension  CollapseDim=2
  Sum of Elements3 : Sum  Inputs=+  CollapseMode=Specified dimension
  Sum of Elements4 : Sum  Inputs=+  CollapseMode=Specified dimension
  Sum of Elements5 : Sum  Inputs=+  CollapseMode=Specified dimension
  Sum1 : Sum  Inputs=|++
  B_r : Outport
  B_theta : Outport  Port=2
  B_phi : Outport  Port=3
  wires:
  dP_matrix/1 -> Matrix Multiply7/1
  r/1 -> Divide/2
  Sum of Elements1/1 -> Matrix Multiply8/1  "Square Bracket"
  Gain3/1 -> Divide1/1
  Sum1/1 -> Matrix Multiply11/2
  Power/1 -> Matrix Multiply14/2, Matrix Multiply8/2, Matrix Multiply5/1
  Matrix Multiply9/1 -> Sum1/1
  SinCos/1 -> Matrix Multiply/2
  SinCos/2 -> Matrix Multiply1/2
  Matrix Multiply5/1 -> Matrix Multiply6/2
  Matrix Multiply/1 -> Matrix Multiply9/1, Matrix Multiply3/2  "5x6 matrix with sin(m*phi) on rows"
  Constant2/1 -> Matrix Multiply10/2, Matrix Multiply3/1
  Constant1/1 -> Matrix Multiply1/1, Matrix Multiply/1
  Constant/1 -> Matrix Multiply2/2, Gain2/1
  Gain/1 -> B_theta/1  "B_theta"
  Matrix Multiply4/1 -> Sum of Elements/1
  Longitude/1 -> Gain1/1
  Matrix Multiply11/1 -> Sum of Elements2/1
  Sum of Elements5/1 -> Gain3/1
  Earth radius/1 -> Divide/1
  Gain1/1 -> SinCos/1
  Divide/1 -> Power/1
  colatitude/1 -> Sin/1
  Matrix Multiply7/1 -> Sum of Elements1/1
  Divide1/1 -> B_phi/1
  Matrix Multiply14/1 -> Sum of Elements5/1
  Matrix Multiply8/1 -> Sum of Elements4/1
  Sum of Elements/1 -> Matrix Multiply6/1  "Square Bracket"
  Matrix Multiply1/1 -> Matrix Multiply10/1, Matrix Multiply2/1  "5x6 matrix with cos(m*phi) on rows"
  Add/1 -> Matrix Multiply7/2, Matrix Multiply4/2
  P_matrix/1 -> Matrix Multiply11/1, Matrix Multiply4/1
  Constant4/1 -> Power/2
  Sin/1 -> Divide1/2
  Constant5/1 -> Matrix Multiply5/2
  Matrix Multiply2/1 -> Add/2
  Sum of Elements4/1 -> Gain/1
  Matrix Multiply6/1 -> Sum of Elements3/1
  Matrix Multiply3/1 -> Add/1
  Gain2/1 -> Matrix Multiply9/2
  Sum of Elements2/1 -> Matrix Multiply14/1  "Square Bracket"
  Matrix Multiply10/1 -> Sum1/2
  Sum of Elements3/1 -> B_r/1  "B_r"

== system satellite_ADCS_pointing_simulation/Disturbance Torques/Magnetic Disturbance Torque n5/Subsystem5 ==
  note: declination
  note: right ascension
  Br : Inport
  Bth : Inport  Port=2
  Bphi : Inport  Port=3
  RA : Inport  Port=4
  DELTA : Inport  Port=5
  Mux : Mux  Inputs=3
  Product{1..8} (8 alike) : Product
  SinCos : Trigonometry  Operator=sincos
  SinCos1 : Trigonometry  Operator=sincos
  Subtract3 : Sum  Inputs=+-
  Subtract4 : Sum  Inputs=+-
  Sum : Sum  Inputs=|++
  Sum1 : Sum  Inputs=|++
  B_N : Outport
  wires:
  SinCos1/2 -> Product8/2, Product1/2  "cosD"
  RA/1 -> SinCos/1
  Sum1/1 -> Mux/2  "B2"
  Br/1 -> Product7/1, Product1/1
  Bth/1 -> Product8/1, Product2/1
  Product5/1 -> Sum1/1
  SinCos/2 -> Product6/2, Product3/2  "cosA"
  Bphi/1 -> Product4/1, Product6/1
  Product8/1 -> Subtract4/2
  Product3/1 -> Subtract3/1
  SinCos/1 -> Product5/2, Product4/2  "sinA"
  Product7/1 -> Subtract4/1
  SinCos1/1 -> Product7/2, Product2/2  "sinD"
  Product4/1 -> Subtract3/2
  Subtract3/1 -> Mux/1  "B1"
  Sum/1 -> Product5/1, Product3/1
  Product6/1 -> Sum1/2
  Subtract4/1 -> Mux/3  "B3"
  Product1/1 -> Sum/1
  Product2/1 -> Sum/2
  Mux/1 -> B_N/1
  DELTA/1 -> SinCos1/1

== system satellite_ADCS_pointing_simulation/Euler Angles Kinematics/312 kin/EA ==
  A : Inport
  13 : Selector  NumberOfDimensions=2  InputPortWidth=3  IndexOptions=Index vector (dialog),Index vector (dialog)  Indices=1,3  OutputSizes=1,1
  21 : Selector  NumberOfDimensions=2  InputPortWidth=3  IndexOptions=Index vector (dialog),Index vector (dialog)  Indices=2,1  OutputSizes=1,1
  22 : Selector  NumberOfDimensions=2  InputPortWidth=3  IndexOptions=Index vector (dialog),Index vector (dialog)  Indices=2,2  OutputSizes=1,1
  23 : Selector  NumberOfDimensions=2  InputPortWidth=3  IndexOptions=Index vector (dialog),Index vector (dialog)  Indices=2,3  OutputSizes=1,1
  33 : Selector  NumberOfDimensions=2  InputPortWidth=3  IndexOptions=Index vector (dialog),Index vector (dialog)  Indices=3,3  OutputSizes=1,1
  Asin : Trigonometry  Operator=asin
  Atan1 : Trigonometry  Operator=atan2
  Atan2 : Trigonometry  Operator=atan2
  Gain : Gain  Gain=-1
  Gain1 : Gain  Gain=-1
  Mux : Mux  Inputs=3
  EA312 : Outport
  wires:
  A/1 -> 23/1, 22/1, 21/1, 33/1, 13/1
  23/1 -> Asin/1
  13/1 -> Gain/1
  33/1 -> Atan2/2
  21/1 -> Gain1/1
  22/1 -> Atan1/2
  Asin/1 -> Mux/2  "th"
  Atan2/1 -> Mux/3  "psi"
  Atan1/1 -> Mux/1  "phi"
  Mux/1 -> EA312/1
  Gain/1 -> Atan2/1
  Gain1/1 -> Atan1/1

== system satellite_ADCS_pointing_simulation/Euler Angles Kinematics/312 kin/Logic Switch 312 ==
  note: singularity check
  note: tollranza 10°
  EA : Inport
  Abs1 : Abs  SaturateOnIntegerOverflow=off
  Add6 : Sum  Inputs=+-
  Add7 : Sum  Inputs=-+
  Constant2 : Constant  Value=1/2
  Constant4 : Constant  Value=0.056
  Gain2 : Gain  Gain=1/pi
  GreaterThan : RelationalOperator  OutDataTypeStr=boolean  RndMeth=Simplest  InputSameDT=off
  Round : Rounding  Operator=round
  Scope : Scope
  Selector4 : Selector  InputPortWidth=3  IndexOptions=Index vector (dialog)  Indices=2  OutputSizes=1
  Enable : Outport
  wires:
  Add6/1 -> Abs1/1  "th/pi-n"
  Gain2/1 -> Add7/2  "th/pi"
  Selector4/1 -> Gain2/1  "theta"
  Add7/1 -> Add6/1, Round/1  "th/pi-1/2"
  Constant2/1 -> Add7/1
  Constant4/1 -> GreaterThan/2
  Round/1 -> Add6/2  "n"
  Abs1/1 -> GreaterThan/1
  EA/1 -> Selector4/1  "EA"
  GreaterThan/1 -> Scope/1, Enable/1  "Enable"

== system satellite_ADCS_pointing_simulation/Euler Angles Kinematics/312 kin/R312 ==
  EA312 : Inport
  Demux : Demux  Outputs=3
  Matrix Multiply : Product  Inputs=3  Multiplication=Matrix(*)
  R1 : Subsystem
  R2 : Subsystem
  R3 : Subsystem
  Transpose : Math  Operator=transpose
  R312 : Outport
  wires:
  EA312/1 -> Demux/1
  Demux/1 -> R3/1(a)
  Demux/2 -> R1/1(a)
  Demux/3 -> R2/1(a)
  R1/1(R1) -> Matrix Multiply/2
  R3/1(R3) -> Matrix Multiply/1
  R2/1(R2) -> Matrix Multiply/3
  Matrix Multiply/1 -> Transpose/1
  Transpose/1 -> R312/1

== system satellite_ADCS_pointing_simulation/Euler Angles Kinematics/312 kin/R313 ==
  EA313 : Inport
  Demux : Demux  Outputs=3
  Matrix Multiply : Product  Inputs=3  Multiplication=Matrix(*)
  R1 : Subsystem
  R3 : Subsystem
  R3' : Subsystem
  Transpose : Math  Operator=transpose
  R313 : Outport
  wires:
  EA313/1 -> Demux/1
  Demux/1 -> R3/1(a)
  Demux/2 -> R1/1(a)
  Demux/3 -> R3'/1(a)
  R1/1(R1) -> Matrix Multiply/2
  R3/1(R3) -> Matrix Multiply/1
  R3'/1(R3) -> Matrix Multiply/3
  Matrix Multiply/1 -> Transpose/1
  Transpose/1 -> R313/1

== system satellite_ADCS_pointing_simulation/Euler Angles Kinematics/313 kin/EA313 ==
  A : Inport
  13 : Selector  NumberOfDimensions=2  InputPortWidth=3  IndexOptions=Index vector (dialog),Index vector (dialog)  Indices=1,3  OutputSizes=1,1
  23 : Selector  NumberOfDimensions=2  InputPortWidth=3  IndexOptions=Index vector (dialog),Index vector (dialog)  Indices=2,3  OutputSizes=1,1
  31 : Selector  NumberOfDimensions=2  InputPortWidth=3  IndexOptions=Index vector (dialog),Index vector (dialog)  Indices=3,1  OutputSizes=1,1
  32 : Selector  NumberOfDimensions=2  InputPortWidth=3  IndexOptions=Index vector (dialog),Index vector (dialog)  Indices=3,2  OutputSizes=1,1
  33 : Selector  NumberOfDimensions=2  InputPortWidth=3  IndexOptions=Index vector (dialog),Index vector (dialog)  Indices=3,3  OutputSizes=1,1
  Asin : Trigonometry  Operator=acos
  Atan1 : Trigonometry  Operator=atan2
  Atan2 : Trigonometry  Operator=atan2
  Gain : Gain  Gain=-1
  Mux : Mux  Inputs=3
  EA313 : Outport
  wires:
  A/1 -> 31/1, 32/1, 33/1, 23/1, 13/1
  33/1 -> Asin/1
  31/1 -> Atan2/1
  32/1 -> Gain/1
  13/1 -> Atan1/1
  23/1 -> Atan1/2
  Asin/1 -> Mux/2  "th"
  Atan2/1 -> Mux/1  "phi"
  Atan1/1 -> Mux/3  "psi"
  Mux/1 -> EA313/1
  Gain/1 -> Atan2/2  "phi"

== system satellite_ADCS_pointing_simulation/Euler Angles Kinematics/313 kin/Logic Switch 313 ==
  note: singularity check
  note: tollranza 10°
  EA : Inport
  Abs1 : Abs  SaturateOnIntegerOverflow=off
  Add6 : Sum  Inputs=+-
  Constant4 : Constant  Value=0.056
  Gain2 : Gain  Gain=1/pi
  GreaterThan : RelationalOperator  OutDataTypeStr=boolean  RndMeth=Simplest  InputSameDT=off
  Round : Rounding  Operator=round
  Scope : Scope
  Selector4 : Selector  InputPortWidth=3  IndexOptions=Index vector (dialog)  Indices=2  OutputSizes=1
  Enable : Outport
  wires:
  Add6/1 -> Abs1/1  "th/pi-n"
  Gain2/1 -> Round/1, Add6/1  "th/pi"
  Selector4/1 -> Gain2/1  "theta"
  Constant4/1 -> GreaterThan/2
  Round/1 -> Add6/2  "n"
  Abs1/1 -> GreaterThan/1
  EA/1 -> Selector4/1  "EA"
  GreaterThan/1 -> Scope/1, Enable/1  "Enable"

== system satellite_ADCS_pointing_simulation/Euler Angles Kinematics/313 kin/R312 ==
  EA312 : Inport
  Demux : Demux  Outputs=3
  Matrix Multiply : Product  Inputs=3  Multiplication=Matrix(*)
  R1 : Subsystem
  R2 : Subsystem
  R3 : Subsystem
  Transpose : Math  Operator=transpose
  R312 : Outport
  wires:
  EA312/1 -> Demux/1
  Demux/1 -> R3/1(a)
  Demux/2 -> R1/1(a)
  Demux/3 -> R2/1(a)
  R1/1(R1) -> Matrix Multiply/2
  R3/1(R3) -> Matrix Multiply/1
  R2/1(R2) -> Matrix Multiply/3
  Matrix Multiply/1 -> Transpose/1
  Transpose/1 -> R312/1

== system satellite_ADCS_pointing_simulation/Euler Angles Kinematics/313 kin/R313 ==
  EA312 : Inport
  Demux : Demux  Outputs=3
  Matrix Multiply : Product  Inputs=3  Multiplication=Matrix(*)
  R1 : Subsystem
  R3 : Subsystem
  R3' : Subsystem
  Transpose : Math  Operator=transpose
  R313 : Outport
  wires:
  EA312/1 -> Demux/1
  Demux/1 -> R3/1(a)
  Demux/2 -> R1/1(a)
  Demux/3 -> R3'/1(a)
  R1/1(R1) -> Matrix Multiply/2
  R3/1(R3) -> Matrix Multiply/1
  R3'/1(R3) -> Matrix Multiply/3
  Matrix Multiply/1 -> Transpose/1
  Transpose/1 -> R313/1

== system satellite_ADCS_pointing_simulation/SAD/Attitude Determination/Algebraic Attitude Determination ==
  note: Attitude Determination
  S : Inport
  V : Inport  Port=2
  E : Inport  Port=3
  "1 for 3s Method 0 for 2s Method " : Scope
  2s Method : Subsystem  TreatAsAtomicUnit=on
  3s Method : Subsystem  TreatAsAtomicUnit=on
  Constant : Constant  Value=3
  Equal : RelationalOperator  Operator===  OutDataTypeStr=boolean  RndMeth=Simplest  InputSameDT=off
  Merge : Merge
  NOT : Logic  Operator=NOT  AllPortsSameDT=off  OutDataTypeStr=boolean
  Sum of Elements : Sum  Inputs=+
  A_b/n : Outport
  wires:
  NOT/1 -> 2s Method/Enable
  Equal/1 -> 3s Method/Enable, NOT/1, "1 for 3s Method 0 for 2s Method "/1
  Constant/1 -> Equal/1
  Sum of Elements/1 -> Equal/2
  E/1 -> Sum of Elements/1, 2s Method/3(E)
  Merge/1 -> A_b/n/1
  2s Method/1(A_b/n) -> Merge/2
  V/1 -> 2s Method/2(V), 3s Method/2(V)
  S/1 -> 3s Method/1(S), 2s Method/1(S)
  3s Method/1(A_b/n) -> Merge/1

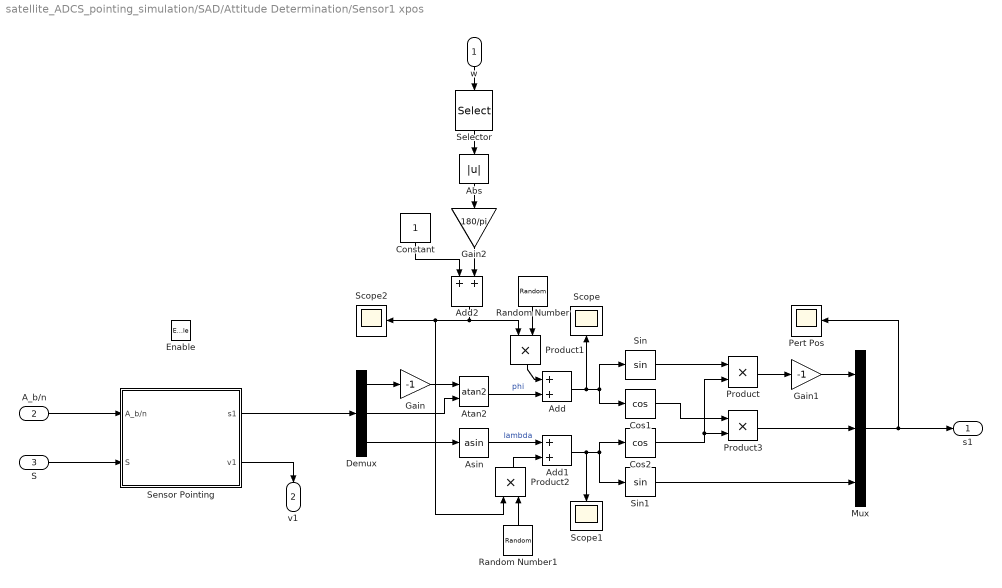
== system satellite_ADCS_pointing_simulation/SAD/Attitude Determination/Sensor1 xpos ==
  w : Inport
  A_b/n : Inport  Port=2
  S : Inport  Port=3
  Enable : EnablePort  PropagateVarSize=During execution
  Abs : Abs  SaturateOnIntegerOverflow=off
  Add : Sum
  Add1 : Sum
  Add2 : Sum
  Asin : Trigonometry  Operator=asin
  Atan2 : Trigonometry  Operator=atan2
  Constant : Constant
  Cos1 : Trigonometry  Operator=cos
  Cos2 : Trigonometry  Operator=cos
  Demux : Demux  Outputs=3
  Gain : Gain  Gain=-1
  Gain1 : Gain  Gain=-1
  Gain2 : Gain  Gain=180/pi
  Mux : Mux  Inputs=3
  Pert Pos : Scope
  Product{,1..3} (4 alike) : Product
  Random Number : RandomNumber  Variance=sensor_noise^2  SampleTime=sensor_sample_time
  Random Number1 : RandomNumber  Variance=sensor_noise^2  SampleTime=sensor_sample_time
  Scope : Scope
  Scope1 : Scope
  Scope2 : Scope
  Selector : Selector  InputPortWidth=3  IndexOptions=Index vector (dialog)  Indices=1  OutputSizes=1
  Sensor Pointing : Subsystem
  Sin : Trigonometry
  Sin1 : Trigonometry
  s1 : Outport
  v1 : Outport  Port=2
  wires:
  Sensor Pointing/2(v1) -> v1/1
  Sensor Pointing/1(s1) -> Demux/1
  S/1 -> Sensor Pointing/2(S)
  A_b/n/1 -> Sensor Pointing/1(A_b/n)
  Add/1 -> Scope/1, Sin/1, Cos1/1
  Asin/1 -> Add1/1  "lambda"
  Product2/1 -> Add1/2
  Demux/1 -> Gain/1
  Atan2/1 -> Add/2  "phi"
  Demux/2 -> Atan2/2
  Cos2/1 -> Product3/2, Product/2
  Gain/1 -> Atan2/1
  Add1/1 -> Cos2/1, Sin1/1, Scope1/1
  Sin1/1 -> Mux/3
  Gain1/1 -> Mux/1
  Sin/1 -> Product/1
  Mux/1 -> Pert Pos/1, s1/1
  Demux/3 -> Asin/1
  Cos1/1 -> Product3/1
  Product/1 -> Gain1/1
  Product3/1 -> Mux/2
  Product1/1 -> Add/1
  w/1 -> Selector/1
  Gain2/1 -> Add2/2
  Selector/1 -> Abs/1
  Random Number/1 -> Product1/2
  Add2/1 -> Product1/1, Product2/1, Scope2/1
  Random Number1/1 -> Product2/2
  Abs/1 -> Gain2/1
  Constant/1 -> Add2/1

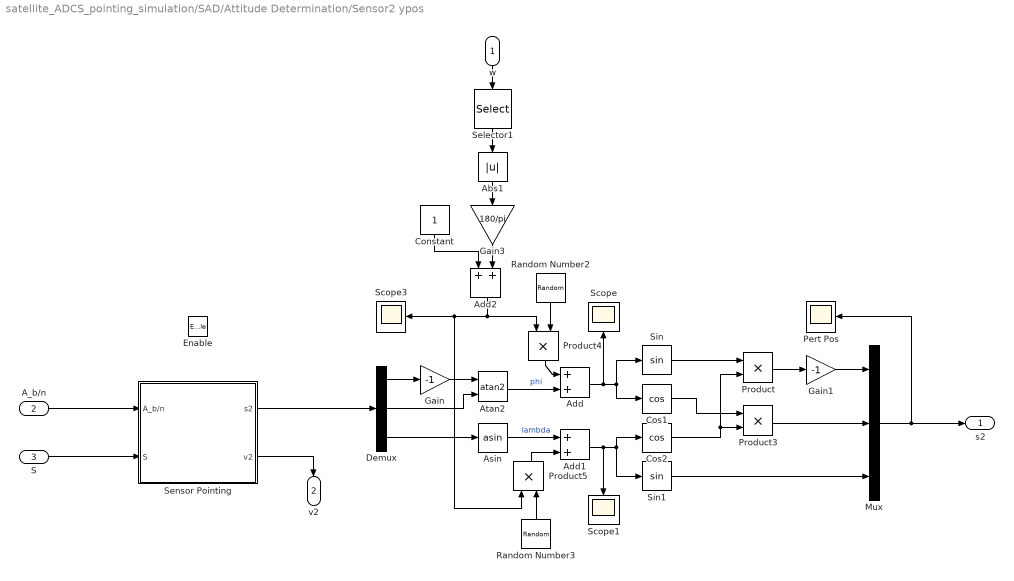
== system satellite_ADCS_pointing_simulation/SAD/Attitude Determination/Sensor2 ypos ==
  w : Inport
  A_b/n : Inport  Port=2
  S : Inport  Port=3
  Enable : EnablePort  PropagateVarSize=During execution
  Abs1 : Abs  SaturateOnIntegerOverflow=off
  Add : Sum
  Add1 : Sum
  Add2 : Sum
  Asin : Trigonometry  Operator=asin
  Atan2 : Trigonometry  Operator=atan2
  Constant : Constant
  Cos1 : Trigonometry  Operator=cos
  Cos2 : Trigonometry  Operator=cos
  Demux : Demux  Outputs=3
  Gain : Gain  Gain=-1
  Gain1 : Gain  Gain=-1
  Gain3 : Gain  Gain=180/pi
  Mux : Mux  Inputs=3
  Pert Pos : Scope
  Product{,3..5} (4 alike) : Product
  Random Number2 : RandomNumber  Variance=sensor_noise^2  SampleTime=sensor_sample_time
  Random Number3 : RandomNumber  Variance=sensor_noise^2  SampleTime=sensor_sample_time
  Scope : Scope
  Scope1 : Scope
  Scope3 : Scope
  Selector1 : Selector  InputPortWidth=3  IndexOptions=Index vector (dialog)  Indices=2  OutputSizes=1
  Sensor Pointing : Subsystem
  Sin : Trigonometry
  Sin1 : Trigonometry
  s2 : Outport
  v2 : Outport  Port=2
  wires:
  Sensor Pointing/2(v2) -> v2/1
  Sensor Pointing/1(s2) -> Demux/1
  S/1 -> Sensor Pointing/2(S)
  A_b/n/1 -> Sensor Pointing/1(A_b/n)
  Gain1/1 -> Mux/1
  Sin1/1 -> Mux/3
  Mux/1 -> Pert Pos/1, s2/1
  Demux/3 -> Asin/1
  Product3/1 -> Mux/2
  Cos1/1 -> Product3/1
  Gain/1 -> Atan2/1
  Product/1 -> Gain1/1
  Sin/1 -> Product/1
  Add1/1 -> Cos2/1, Sin1/1, Scope1/1
  Cos2/1 -> Product3/2, Product/2
  Atan2/1 -> Add/2  "phi"
  Asin/1 -> Add1/1  "lambda"
  Demux/2 -> Atan2/2
  Add/1 -> Scope/1, Sin/1, Cos1/1
  Demux/1 -> Gain/1
  Product4/1 -> Add/1
  Product5/1 -> Add1/2
  w/1 -> Selector1/1
  Random Number2/1 -> Product4/2
  Add2/1 -> Product4/1, Scope3/1, Product5/1
  Selector1/1 -> Abs1/1
  Random Number3/1 -> Product5/2
  Abs1/1 -> Gain3/1
  Constant/1 -> Add2/1
  Gain3/1 -> Add2/2

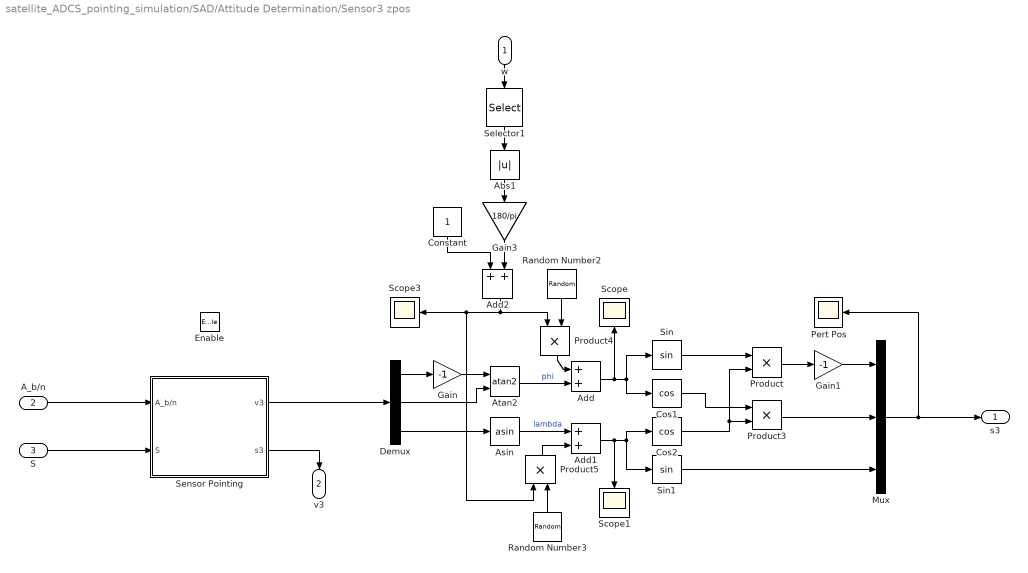
== system satellite_ADCS_pointing_simulation/SAD/Attitude Determination/Sensor3 zpos ==
  w : Inport
  A_b/n : Inport  Port=2
  S : Inport  Port=3
  Enable : EnablePort  PropagateVarSize=During execution
  Abs1 : Abs  SaturateOnIntegerOverflow=off
  Add : Sum
  Add1 : Sum
  Add2 : Sum
  Asin : Trigonometry  Operator=asin
  Atan2 : Trigonometry  Operator=atan2
  Constant : Constant
  Cos1 : Trigonometry  Operator=cos
  Cos2 : Trigonometry  Operator=cos
  Demux : Demux  Outputs=3
  Gain : Gain  Gain=-1
  Gain1 : Gain  Gain=-1
  Gain3 : Gain  Gain=180/pi
  Mux : Mux  Inputs=3
  Pert Pos : Scope
  Product{,3..5} (4 alike) : Product
  Random Number2 : RandomNumber  Variance=sensor_noise^2  SampleTime=sensor_sample_time
  Random Number3 : RandomNumber  Variance=sensor_noise^2  SampleTime=sensor_sample_time
  Scope : Scope
  Scope1 : Scope
  Scope3 : Scope
  Selector1 : Selector  InputPortWidth=3  IndexOptions=Index vector (dialog)  Indices=3  OutputSizes=1
  Sensor Pointing : Subsystem
  Sin : Trigonometry
  Sin1 : Trigonometry
  s3 : Outport
  v3 : Outport  Port=2
  wires:
  Sensor Pointing/2(s3) -> v3/1
  Sensor Pointing/1(v3) -> Demux/1
  S/1 -> Sensor Pointing/2(S)
  A_b/n/1 -> Sensor Pointing/1(A_b/n)
  Gain1/1 -> Mux/1
  Sin1/1 -> Mux/3
  Mux/1 -> Pert Pos/1, s3/1
  Demux/3 -> Asin/1
  Product3/1 -> Mux/2
  Cos1/1 -> Product3/1
  Gain/1 -> Atan2/1
  Product/1 -> Gain1/1
  Sin/1 -> Product/1
  Add1/1 -> Cos2/1, Sin1/1, Scope1/1
  Cos2/1 -> Product3/2, Product/2
  Atan2/1 -> Add/2  "phi"
  Asin/1 -> Add1/1  "lambda"
  Demux/2 -> Atan2/2
  Add/1 -> Scope/1, Sin/1, Cos1/1
  Demux/1 -> Gain/1
  Product4/1 -> Add/1
  Product5/1 -> Add1/2
  w/1 -> Selector1/1
  Random Number2/1 -> Product4/2
  Add2/1 -> Product4/1, Scope3/1, Product5/1
  Selector1/1 -> Abs1/1
  Random Number3/1 -> Product5/2
  Abs1/1 -> Gain3/1
  Constant/1 -> Add2/1
  Gain3/1 -> Add2/2

== system satellite_ADCS_pointing_simulation/SAD/Attitude Determination/Sun Sensors ==
  S_n : Inport
  A_b/n : Inport  Port=2
  Mux : Mux  Inputs=3
  Sun Sensor xpos : Subsystem
  Sun Sensor ypos : Subsystem
  Sun Sensor zpos : Subsystem
  Sun Obstruction : Outport
  wires:
  Mux/1 -> Sun Obstruction/1
  Sun Sensor zpos/1(s3) -> Mux/3
  Sun Sensor xpos/1(s1) -> Mux/1
  Sun Sensor ypos/1(s2) -> Mux/2
  S_n/1 -> Sun Sensor ypos/2(S_n), Sun Sensor zpos/2(S_n), Sun Sensor xpos/2(S_n)
  A_b/n/1 -> Sun Sensor ypos/1(A_b/n), Sun Sensor zpos/1(A_b/n), Sun Sensor xpos/1(A_b/n)

== system satellite_ADCS_pointing_simulation/SAD/Attitude Determination/Wabha Attitude Determination ==
  s1 : Inport
  v1 : Inport  Port=2
  s2 : Inport  Port=3
  v2 : Inport  Port=4
  s3 : Inport  Port=5
  v3 : Inport  Port=6
  E : Inport  Port=7
  If : If  IfExpression=u1 == 3
  Merge : Merge
  Scope : Scope
  Sum of Elements : Sum  Inputs=+
  Wabha Attitude Determination 2s : Subsystem
  Wabha Attitude Determination 3s : Subsystem
  A*_b/n : Outport
  wires:
  v3/1 -> Wabha Attitude Determination 2s/7(v3), Wabha Attitude Determination 3s/6(v3)
  s3/1 -> Wabha Attitude Determination 2s/6(s3), Wabha Attitude Determination 3s/5(s3)
  v2/1 -> Wabha Attitude Determination 2s/5(v2), Wabha Attitude Determination 3s/4(v2)
  s2/1 -> Wabha Attitude Determination 2s/4(s2), Wabha Attitude Determination 3s/3(s2)
  v1/1 -> Wabha Attitude Determination 2s/3(v1), Wabha Attitude Determination 3s/2(v1)
  s1/1 -> Wabha Attitude Determination 2s/2(s1), Wabha Attitude Determination 3s/1(s1)
  Merge/1 -> A*_b/n/1
  If/1 -> Wabha Attitude Determination 3s/Action
  Wabha Attitude Determination 2s/1(A*_b/n) -> Merge/1
  If/2 -> Wabha Attitude Determination 2s/Action
  E/1 -> Sum of Elements/1, Wabha Attitude Determination 2s/1(E)
  Wabha Attitude Determination 3s/1(A*_b/n) -> Merge/2
  Sum of Elements/1 -> If/1, Scope/1

== system satellite_ADCS_pointing_simulation/Euler Angles Kinematics/312 kin/R312/R1 ==
  a : Inport
  Add : Sum  Inputs=+++
  Constant : Constant  Value=[0 0 0; 0 1 0; 0 0 1]
  Constant1 : Constant  Value=[0 0 0; 0 0 -1; 0 1 0]
  Constant2 : Constant  Value=[1 0 0; 0 0 0; 0 0 0]
  Cos : Trigonometry  Operator=cos
  Product : Product
  Product1 : Product
  Sin : Trigonometry
  R1 : Outport
  wires:
  a/1 -> Cos/1, Sin/1
  Cos/1 -> Product/2
  Constant/1 -> Product/1
  Constant1/1 -> Product1/1
  Sin/1 -> Product1/2
  Product/1 -> Add/1
  Constant2/1 -> Add/3
  Product1/1 -> Add/2
  Add/1 -> R1/1

== system satellite_ADCS_pointing_simulation/Euler Angles Kinematics/312 kin/R312/R2 ==
  a : Inport
  Add : Sum  Inputs=+++
  Constant : Constant  Value=[1 0 0; 0 0 0; 0 0 1]
  Constant1 : Constant  Value=[0 0 1; 0 0 0; -1 0 0]
  Constant2 : Constant  Value=[0 0 0; 0 1 0; 0 0 0]
  Cos : Trigonometry  Operator=cos
  Product : Product
  Product1 : Product
  Sin : Trigonometry
  R2 : Outport
  wires:
  a/1 -> Cos/1, Sin/1
  Cos/1 -> Product/2
  Constant/1 -> Product/1
  Constant1/1 -> Product1/1
  Sin/1 -> Product1/2
  Product/1 -> Add/1
  Constant2/1 -> Add/3
  Product1/1 -> Add/2
  Add/1 -> R2/1

== system satellite_ADCS_pointing_simulation/Euler Angles Kinematics/312 kin/R312/R3 ==
  a : Inport
  Add : Sum  Inputs=+++
  Constant : Constant  Value=[1 0 0; 0 1 0; 0 0 0]
  Constant1 : Constant  Value=[0 -1 0; 1 0 0; 0 0 0]
  Constant2 : Constant  Value=[0 0 0; 0 0 0; 0 0 1]
  Cos : Trigonometry  Operator=cos
  Product : Product
  Product1 : Product
  Sin : Trigonometry
  R3 : Outport
  wires:
  a/1 -> Cos/1, Sin/1
  Cos/1 -> Product/2
  Constant/1 -> Product/1
  Constant1/1 -> Product1/1
  Sin/1 -> Product1/2
  Product/1 -> Add/1
  Constant2/1 -> Add/3
  Product1/1 -> Add/2
  Add/1 -> R3/1

== system satellite_ADCS_pointing_simulation/Euler Angles Kinematics/312 kin/R313/R1 ==
  a : Inport
  Add : Sum  Inputs=+++
  Constant : Constant  Value=[0 0 0; 0 1 0; 0 0 1]
  Constant1 : Constant  Value=[0 0 0; 0 0 -1; 0 1 0]
  Constant2 : Constant  Value=[1 0 0; 0 0 0; 0 0 0]
  Cos : Trigonometry  Operator=cos
  Product : Product
  Product1 : Product
  Sin : Trigonometry
  R1 : Outport
  wires:
  a/1 -> Cos/1, Sin/1
  Cos/1 -> Product/2
  Constant/1 -> Product/1
  Constant1/1 -> Product1/1
  Sin/1 -> Product1/2
  Product/1 -> Add/1
  Constant2/1 -> Add/3
  Product1/1 -> Add/2
  Add/1 -> R1/1
